simulink library "bamFsm"  (R2023b)
settings: Solver=VariableStepAuto  StartTime=0.0  StopTime=10.0  RelTol=1e-3
settings Model: Creator=Professional  LastModifiedBy=zon07
settings SFSimCC: SimTargetLang=C++

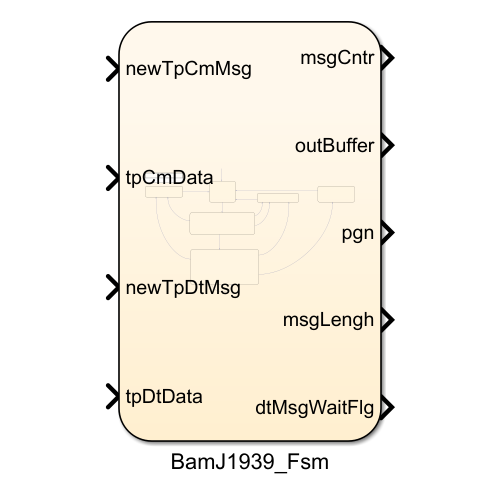
[thumbnail: Simulink's stored preview of the top-level diagram]
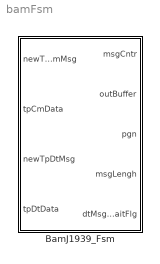
== system bamFsm ==
  BamJ1939_Fsm : Stateflow chart  TreatAsAtomicUnit=on
      settings: PortSchema="{\"entries\":[{\"content\":{\"sides\":[{\"content\":{\"connectorIds\":[\"In3\",\"In1\",\"In4\",\"In2\"]},\"type\":\"ConnectorPlacement.EquallySpacedRectSide\",\"uuid\":\"f0437618-7372-46d8-9ab7-ff8929e6fb67\"},{\"content\":{\"connectorIds\":[\"Out2\",\"Out1\",\"Out3\",\"Out4\",\"Out5\"],\"side\":\"RIGHT\"},\"type\":\"ConnectorPlacement.EquallySpacedRectSide\",\"uuid\":\"0536630b-4cc4-4e97-9664-ff8fdcddfe97\"},{\"content\":{\"side\":\"TOP\"},\"type\":\"ConnectorPlacement.EquallySpacedRectSide\",\"uuid\":\"62369740-83f5-4f7d-ae2b-bf987bd5a7ae\"}]},\"type\":\"ConnectorPlacement.EquallySpacedConnector\",\"uuid\":\"7025f99e-73e8-416b-8734-672140f8b319\"}],\"packageUris\":[\"http://schema.mathworks.com/mf0/Connector/R2020b\"],\"version\":\"1.0\"}"

== stateflow chart bamFsm/BamJ1939_Fsm ==
  state CM_WAIT
    en:
    pgnOfPackets = 0x4FFFF;
    totalMsgSize = 0;
    totalPackNum = 0;
    nextPacketNum = 0;
    msgCmplt = false;
    dtMsgWaitFlg = false;
  state TP_DATA_READY
    en:
    dtMsgWaitFlg = false;
    msgCmplt = false;
    msgCntr = msgCntr + uint32(1); % New data
    msgLengh = totalMsgSize;
  state TP_TIMEOUT
    en:
    dtMsgWaitFlg = false;
    outBuffer = clearBuffer(outBuffer, buffLengh);
  state TP_ERROR
    en:
    dtMsgWaitFlg = false;
  state BAM_INIT
    en:
    msgLengh = 0;
    totalMsgSize = uint16(tpCmData(2)) + bitshift(uint16(tpCmData(3)), 8);
    totalPackNum = tpCmData(4);
    pgnOfPackets = uint32(tpCmData(6)) + bitshift(uint32(tpCmData(7)), 8) + ...
    bitshift(uint32(tpCmData(8)), 16)
    pgn = pgnOfPackets;
    dtMsgWaitFlg = true;
  state BAM_DT_COLLECT
    en:
    offsetData = 7 * (uint16(tpDtData(1)) - 1);
    i = uint16(1);
    if(tpDtData(1) == totalPackNum)
    for i = uint16(1):uint16(7 - uint16(mod(uint16(tpDtData(1)*7), totalMsgSize)))
    outBuffer(i + offsetData) = tpDtData(i+1);
    end
    msgCmplt = true;
    else
    for i = uint16(1):uint16(7)
    outBuffer(i + offsetData) = tpDtData(i+1);
    end
    nextPacketNum = tpDtData(1) + 1;
    end
  (default) -> CM_WAIT
  TP_DATA_READY -> CM_WAIT
  TP_TIMEOUT -> CM_WAIT
  BAM_DT_COLLECT -> TP_TIMEOUT [order 3] : after(750, msec)
  BAM_INIT -> TP_TIMEOUT [order 2] : after(750, msec)
  TP_ERROR -> CM_WAIT
  CM_WAIT -> BAM_INIT : [newTpCmMsg &&...
      |  tpCmData(1) == 0x20]
  BAM_INIT -> TP_ERROR [order 1] : [totalMsgSize > buffLengh]
  BAM_INIT -> TP_ERROR [order 3] : [tpDtData(1) ~= uint8(1) && ...
      | newTpDtMsg]
  BAM_DT_COLLECT -> TP_DATA_READY [order 2] : [msgCmplt]
  BAM_DT_COLLECT -> TP_ERROR [order 4] : [tpDtData(1) ~= nextPacketNum && newTpDtMsg]
      | {outBuffer = clearBuffer(outBuffer, buffLengh);}
  BAM_INIT -> BAM_DT_COLLECT [order 4] : [tpDtData(1) == uint8(1)  && newTpDtMsg]
  BAM_DT_COLLECT -> BAM_DT_COLLECT [order 1] : [tpDtData(1) == nextPacketNum &&...
      |  newTpDtMsg]
  data: buff function_input; buffSize function_input; buff function_output; tpCmData input uint8 size=8; tpDtData input uint8 size=8; newTpCmMsg input boolean size=1; totalMsgSize local uint16 size=1; totalPackNum local uint8 size=1; pgnOfPackets local uint32 size=1; outBuffer output uint8 size=buffLengh =0xFF; msgCntr output uint32 size=1 =0; buffLengh constant uint16 size=1 =buffSize; nextPacketNum local uint8 size=1; offsetData local uint16 size=1; newTpDtMsg input boolean size=1 =0; pgn output uint32 size=1; i local uint16; msgCmplt local boolean; msgLengh output uint16 =0; dtMsgWaitFlg output boolean
  function buff = clearBuffer(buff, buffSize):
    | function buff = clearBuffer(buff, buffSize)
    |     arguments
    |         buff (:,1) uint8
    |         buffSize uint16
    |     end
    |     for buffIterator = 1:buffSize
    |         buff(buffIterator) = uint8(0xFF);
    |     end
    | end
